simulink model "EV_Hybrid_Energy_Storage_System"  (R2026a)
settings: Solver=VariableStepAuto  StopTime=20
settings Model: Creator=hazal  LastModifiedBy=hazal

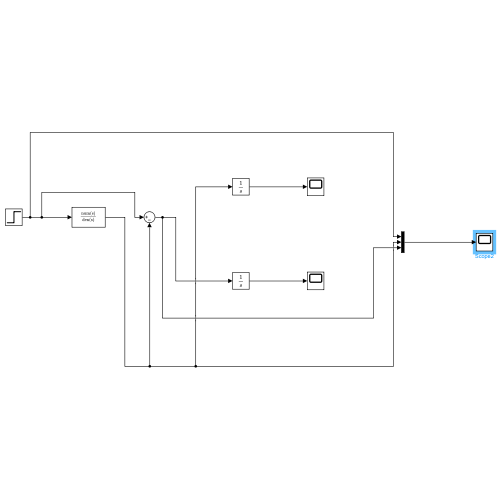
[thumbnail: Simulink's stored preview of the top-level diagram]
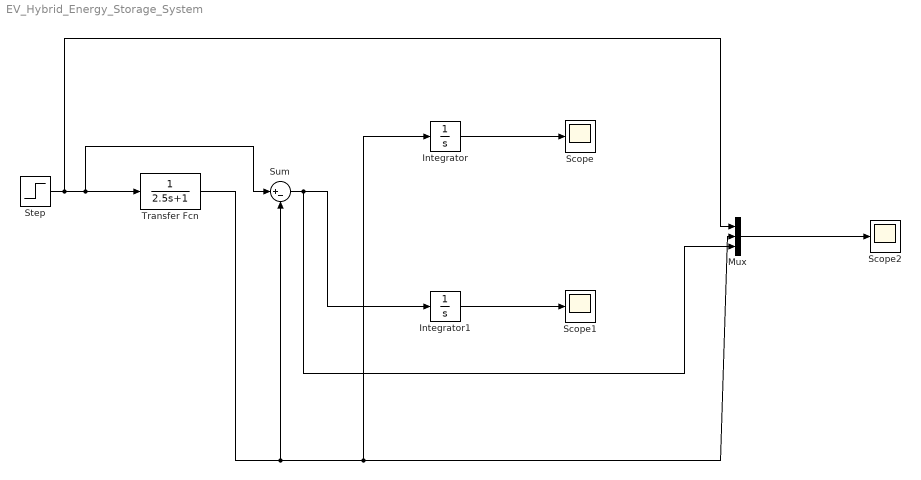
== system EV_Hybrid_Energy_Storage_System ==
  Integrator : Integrator
  Integrator1 : Integrator
  Mux : Mux  Inputs=3
  Scope : Scope
  Scope1 : Scope
  Scope2 : Scope
      settings: ActiveDisplayYMinimum=-9.9999999999999982  ActiveDisplayYMaximum=90  DataLoggingVariableName=ScopeData2
  Step : Step  Time=5  InitialValue=20  FinalValue=80  SampleTime=0
  Sum : Sum  Inputs=|+-
  Transfer Fcn : TransferFcn  Denominator=[2.5 1]
  wires:
  Integrator/1 -> Scope/1
  Integrator1/1 -> Scope1/1
  Transfer Fcn/1 -> Sum/2, Integrator/1, Mux/2
  Sum/1 -> Mux/3, Integrator1/1
  Step/1 -> Mux/1, Sum/1, Transfer Fcn/1
  Mux/1 -> Scope2/1
